simulink model "EReg_Tank_Drainrefusestowork"  (R2025b)
settings: Solver=FixedStepAuto  StartTime=0.0  StopTime=Sim_Duration  FixedStep=1/500  RelTol=1e-3
values from neighbouring files (symbols this model uses):
  A_3 = 13.27e-6    (= 1.327e-05)    [EReg_N2O_Simulink_Init.m]    (also in EReg_Tank_Drain_Init.m = 6e-05)
  Cd_3 = 0.6    [EReg_N2O_Simulink_Init.m]    (also in EReg_Tank_Drain_Init.m = 0.7)
  gamma_N2 = 1.4    [EReg_N2O_Simulink_Init.m]    (also in EReg_Tank_Drain_Init.m; EReg_Tank_Drain_N2O_Sim.m; N2O_Tank_Plant.m)
  K_v_4 = 0.5    [EReg_Tank_Drain_Init.m]
  Kv_1_max = 1.5    [EReg_N2O_Simulink_Init.m]    (also in EReg_Tank_Drain_Init.m = 1; EReg_Tank_Drain_N2O_Sim.m = params.Kv_1_max)
  m_1_0 = rho_1_0 * V_1    (= 2.35097796073)    [EReg_N2O_Simulink_Init.m]    (also in EReg_Tank_Drain_Init.m = 2.2972972973; EReg_Tank_Drain_N2O_Sim.m = params.m_1_0)
  m_2_0 = m_N2_ull_0    [EReg_N2O_Simulink_Init.m]    (also in EReg_Tank_Drain_Init.m = 0.281531531532)
  m_3_0 = m_N2O_liq_0    (= 12)    [EReg_N2O_Simulink_Init.m]    (also in EReg_Tank_Drain_Init.m = 20)
  P_1_0 = 300e5    (= 30000000)    [EReg_N2O_Simulink_Init.m]    (also in EReg_Tank_Drain_Init.m; EReg_Tank_Drain_N2O_Sim.m = params.P_1_0)
  Pst = 101325    [EReg_N2O_Simulink_Init.m]    (also in EReg_Tank_Drain_Init.m)
  R_N2 = 296    [EReg_N2O_Simulink_Init.m]    (also in EReg_Tank_Drain_Init.m; EReg_Tank_Drain_N2O_Sim.m = params.R_N2)
  rho_1_0 = P_1_0 / (R_N2 * T_0_N2)    (= 345.732053049)    [EReg_N2O_Simulink_Init.m]    (also in EReg_Tank_Drain_Init.m = 337.837837838; EReg_Tank_Drain_N2O_Sim.m = m_1_0 / V_1)
  rho_L = rhoL_init    [EReg_N2O_Simulink_Init.m]    (also in EReg_Tank_Drain_Init.m = 1000; EReg_Tank_Drain_N2O_Sim.m = T_to_rhoL(T); EregPlot.m = 1000; N2O_Tank_Plant.m = interp1_lut(T_sat_LUT, rhoL_LUT, T_N2O))
  rhost = Pst / (R_N2 * Tst)    (= 1.25320955222)    [EReg_N2O_Simulink_Init.m]    (also in EReg_Tank_Drain_Init.m)
  servo_off_setpoint = ones(1, Num_Steps)    [EReg_N2O_Simulink_Init.m]    (also in EReg_Tank_Drain_Init.m = zeros(1, Num_Steps))
  T_0_N2 = 293.15    [EReg_N2O_Simulink_Init.m]    (also in EReg_Tank_Drain_Init.m = 300)
  time = linspace(0, Sim_Duration, Num_Steps)    [EReg_N2O_Simulink_Init.m]    (also in EReg_Tank_Drain_Init.m; EReg_Tank_Drain_N2O_Sim.m = (0 : dt : t_end)')
  Tst = 273.15    [EReg_N2O_Simulink_Init.m]    (also in EReg_Tank_Drain_Init.m)
  V_1 = 6.8e-3    (= 0.0068)    [EReg_N2O_Simulink_Init.m]    (also in EReg_Tank_Drain_Init.m; EReg_Tank_Drain_N2O_Sim.m = params.V_1)
  V_2 = 30e-3    (= 0.03)    [EReg_N2O_Simulink_Init.m]    (also in EReg_Tank_Drain_Init.m = 0.025; EReg_Tank_Drain_N2O_Sim.m = params.V_2)
undefined symbols (not defined in the file or in its folder): DiscIntNeverNeededParam
libraries: simulink x2, slpidlib x1
settings Model: Creator=marti  LastModifiedBy=anzashoaib
settings OptimizationCC: ReuseModelBlockBuffer=off
settings RTWCC: GPUComputeCapability=3.5

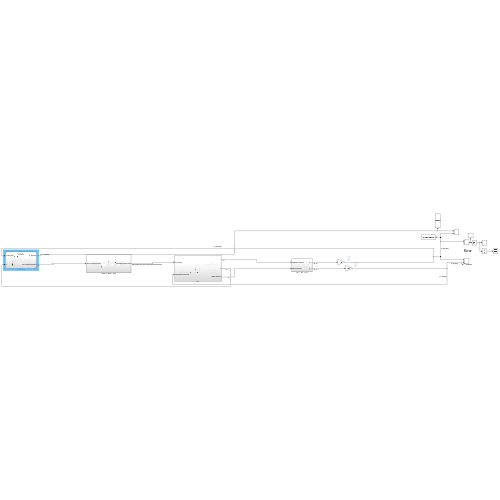
[thumbnail: Simulink's stored preview of the top-level diagram]
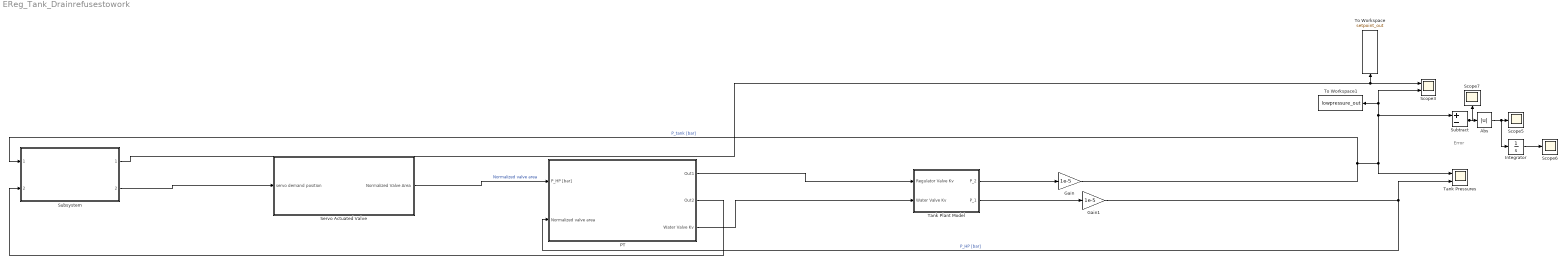
== system EReg_Tank_Drainrefusestowork ==
  note: Error
  Abs : Abs  SaturateOnIntegerOverflow=off
  Gain : Gain  Gain=1e-5
  Gain1 : Gain  Gain=1e-5
  Integrator : Integrator
  "PT " : Subsystem
  Scope3 : Scope  NumInputPorts=2
      settings: ActiveDisplayYMinimum=51.75312  ActiveDisplayYMaximum=64.23854
  Scope5 : Scope
      settings: ActiveDisplayYMinimum=-0.46907  ActiveDisplayYMaximum=4.2216
  Scope6 : Scope
      settings: ActiveDisplayYMinimum=-42.4732  ActiveDisplayYMaximum=382.25884  DataLoggingVariableName=ScopeData2
  Scope7 : Scope
      settings: ActiveDisplayYMinimum=-4.72126  ActiveDisplayYMaximum=4.96726  DataLoggingVariableName=ScopeData3
  Servo Actuated Valve : Subsystem
  Subsystem : Subsystem  ReferencedSubsystem=Controller
  Subtract : Sum  Inputs=+-
  Tank Plant Model : Subsystem
  Tank Pressures : Scope  NumInputPorts=2
      settings: ActiveDisplayYMinimum=22.037093774647268  ActiveDisplayYMaximum=330.88476735837253
  To Workspace : ToWorkspace  VariableName=setpoint_out  SaveFormat=Timeseries  SampleTime=-1
  To Workspace1 : ToWorkspace  VariableName=lowpressure_out  SaveFormat=Timeseries  SampleTime=-1
  wires:
  Tank Plant Model/1(P_2) -> Gain/1
  Tank Plant Model/2(P_1) -> Gain1/1
  Gain/1 -> Subsystem/1, Subtract/1, Scope3/2, To Workspace1/1, Tank Pressures/1  "P_tank [bar]"
  Gain1/1 -> "PT "/2(Normalized valve area), Tank Pressures/2  "P_HP [bar]"
  Subtract/1 -> Scope7/1, Abs/1
  Abs/1 -> Integrator/1, Scope5/1
  Integrator/1 -> Scope6/1
  Subsystem/1 -> To Workspace/1, Scope3/1
  Subsystem/2 -> Servo Actuated Valve/1(servo demand position)
  Servo Actuated Valve/1(Normalized Valve Area) -> "PT "/1(P_HP [bar])  "Normalized valve area"
  "PT "/1(Out1) -> Tank Plant Model/1(Regulator Valve Kv)
  "PT "/2(Out2) -> Subsystem/2
  "PT "/3(Water Valve Kv) -> Tank Plant Model/2(Water Valve Kv)

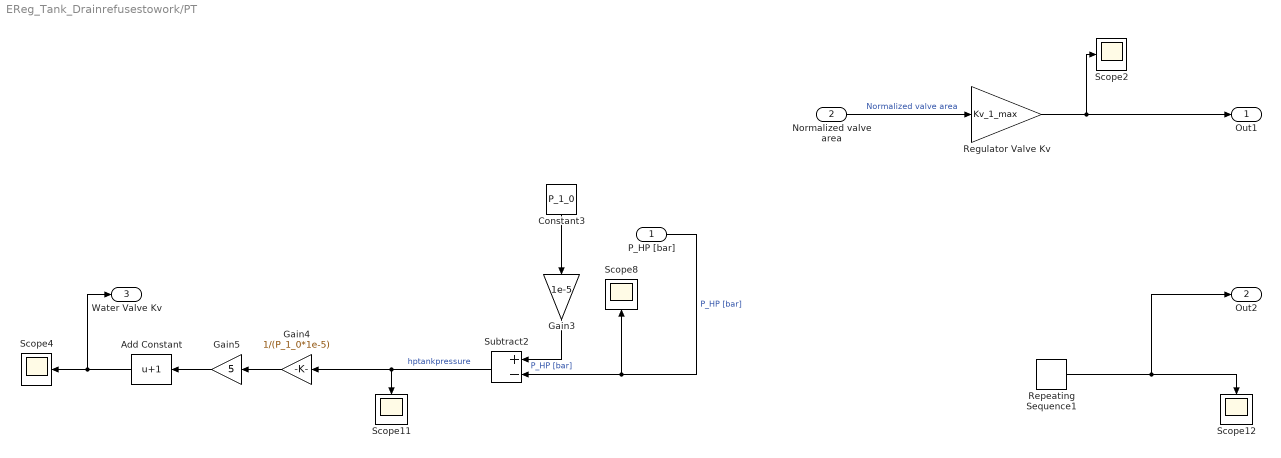
== system EReg_Tank_Drainrefusestowork/PT  ==
  P_HP [bar] : Inport  OutDataTypeStr=double  PortDimensions=1  SampleTime=0
  Normalized valve area : Inport  Port=2  OutDataTypeStr=double  PortDimensions=1  SampleTime=0
  Add Constant : Bias  Bias=1  SaturateOnIntegerOverflow=off
  Constant3 : Constant  Value=P_1_0
  Gain3 : Gain  Gain=1e-5
  Gain4 : Gain  Gain=1/(P_1_0*1e-5)
  Gain5 : Gain  Gain=5
  Regulator Valve Kv : Gain  Gain=Kv_1_max
  Repeating Sequence1 : simulink/Sources/Repeating Sequence  rep_seq_t=time  rep_seq_y=run_valve_setpoint
  Scope{2,4,8,11..12} (5 alike) : Scope
      Scope11 settings: ActiveDisplayYMinimum=-7.98984  ActiveDisplayYMaximum=71.90855  DataLoggingVariableName=ScopeData15
      Scope12 settings: ActiveDisplayYMinimum=-0.125  ActiveDisplayYMaximum=1.125  DataLoggingVariableName=ScopeData16
      Scope2 settings: ActiveDisplayYMinimum=-0.0196  ActiveDisplayYMaximum=0.17636  DataLoggingVariableName=ScopeData17
      Scope4 settings: ActiveDisplayYMinimum=0.86684  ActiveDisplayYMaximum=2.19848  DataLoggingVariableName=ScopeData18
      Scope8 settings: ActiveDisplayYMinimum=229.43787  ActiveDisplayYMaximum=307.84024  DataLoggingVariableName=ScopeData19
  Subtract2 : Sum  Inputs=+-
  Out1 : Outport  OutDataTypeStr=double  PortDimensions=1  SampleTime=0
  Out2 : Outport  Port=2  OutDataTypeStr=double  PortDimensions=1  SampleTime=0
  Water Valve Kv : Outport  Port=3  OutDataTypeStr=double  PortDimensions=1  SampleTime=0
  wires:
  Add Constant/1 -> Water Valve Kv/1, Scope4/1
  Gain3/1 -> Subtract2/1  "P_HP [bar]"
  Gain4/1 -> Gain5/1
  Repeating Sequence1/1 -> Scope12/1, Out2/1
  P_HP [bar]/1 -> Scope8/1, Subtract2/2  "P_HP [bar]"
  Regulator Valve Kv/1 -> Out1/1, Scope2/1
  Constant3/1 -> Gain3/1
  Subtract2/1 -> Gain4/1, Scope11/1  "hptankpressure"
  Gain5/1 -> Add Constant/1
  Normalized valve area/1 -> Regulator Valve Kv/1  "Normalized valve area"

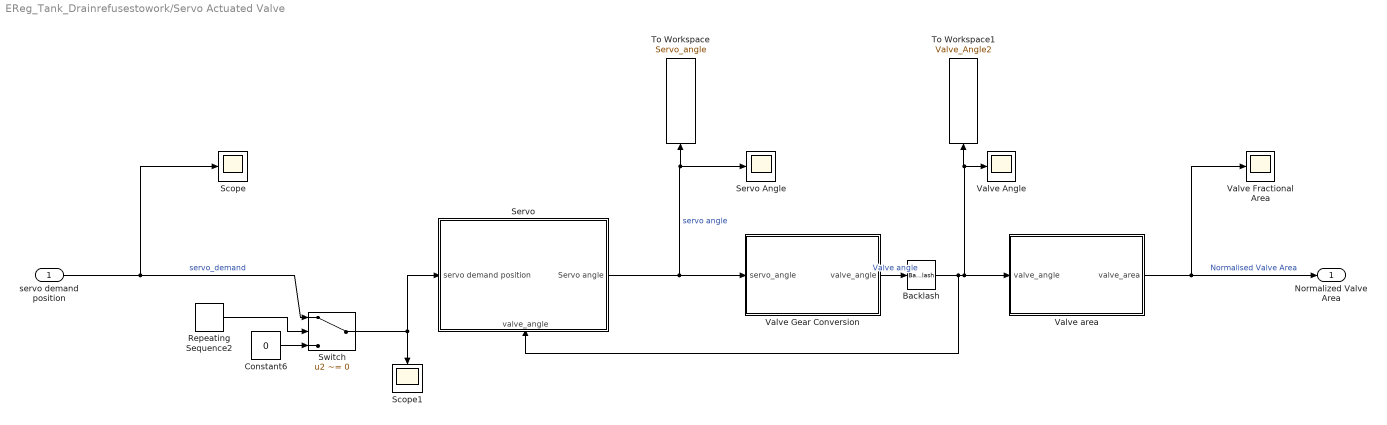
== system EReg_Tank_Drainrefusestowork/Servo Actuated Valve ==
  servo demand position : Inport
  " Valve Gear Conversion" : MATLAB Function  TreatAsAtomicUnit=on
  " Valve area" : MATLAB Function  TreatAsAtomicUnit=on
  Backlash : Backlash  BacklashWidth=0.5  InitialOutput=0.5
  Constant6 : Constant  Value=0
  Repeating Sequence2 : simulink/Sources/Repeating Sequence  rep_seq_t=time(:)  rep_seq_y=servo_off_setpoint(:)
  Scope : Scope
      settings: ActiveDisplayYMinimum=-1660.50954  ActiveDisplayYMaximum=362.9195  DataLoggingVariableName=ScopeData3
  Scope1 : Scope
      settings: ActiveDisplayYMinimum=-1660.50954  ActiveDisplayYMaximum=362.9195  DataLoggingVariableName=ScopeData3
  Servo : Subsystem
      settings: PortSchema="{\"entries\":[{\"content\":{\"sides\":[{\"content\":{\"connectorIds\":[\"In1\"]},\"type\":\"ConnectorPlacement.EquallySpacedRectSide\",\"uuid\":\"80cc8390-5c54-44fd-a47c-7e7786ca55cb\"},{\"content\":{\"connectorIds\":[\"Out1\"],\"side\":\"RIGHT\"},\"type\":\"ConnectorPlacement.EquallySpacedRectSide\",\"uuid\":\"1eac09ca-847a-4c9b-93fa-12e39acf6b4a\"},{\"content\":{\"side\":\"TOP\"},\"type\":\"ConnectorPlacement.EquallySpacedRectSide\",\"uuid\":\"448ec877-4708-4b6f-bd0d-b7e31e141685\"},{\"content\":{\"connectorIds\":[\"In2\"],\"side\":\"BOTTOM\"},\"type\":\"ConnectorPlacement.EquallySpacedRectSide\",\"uuid\":\"b9bb9fb8-2143-4f55-8173-037b619887c5\"}]},\"type\":\"ConnectorPlacement.EquallySpacedConnector\",\"uuid\":\"bf70c898-a427-4eb9-a0e2-218e58098715\"}],\"packageUris\":[\"http://schema.mathworks.com/mf0/Connector/R2020b\"],\"version\":\"1.0\"}"
  Servo Angle : Scope
      settings: ActiveDisplayYMinimum=-2.83907  ActiveDisplayYMaximum=21.23036  DataLoggingVariableName=Servo_Angle  DataLoggingSaveFormat=Array
  Switch : Switch  Criteria=u2 ~= 0  SaturateOnIntegerOverflow=off  InputSameDT=off
  To Workspace : ToWorkspace  VariableName=Servo_angle  SampleTime=-1
      settings: Save2DSignal=2-D array (concatenate along first dimension)
  To Workspace1 : ToWorkspace  VariableName=Valve_Angle2  SampleTime=-1
      settings: Save2DSignal=2-D array (concatenate along first dimension)
  Valve Angle : Scope
      settings: ActiveDisplayYMinimum=-1.35754  ActiveDisplayYMaximum=12.17595  DataLoggingVariableName=Valve_Angle  DataLoggingSaveFormat=Array
  Valve Fractional Area : Scope
      settings: ActiveDisplayYMinimum=-0.0196  ActiveDisplayYMaximum=0.17636  DataLoggingVariableName=ScopeData8
  Normalized Valve Area : Outport
  wires:
  " Valve area"/1(valve_area) -> Normalized Valve Area/1, Valve Fractional Area/1  "Normalised Valve Area"
  " Valve Gear Conversion"/1(valve_angle) -> Backlash/1  "Valve angle"
  servo demand position/1 -> Scope/1, Switch/1  "servo_demand"
  Servo/1(Servo angle) -> " Valve Gear Conversion"/1(servo_angle), To Workspace/1, Servo Angle/1  "servo angle"
  Repeating Sequence2/1 -> Switch/2
  Constant6/1 -> Switch/3
  Switch/1 -> Servo/1(servo demand position), Scope1/1
  Backlash/1 -> " Valve area"/1(valve_angle), To Workspace1/1, Valve Angle/1, Servo/2(valve_angle)

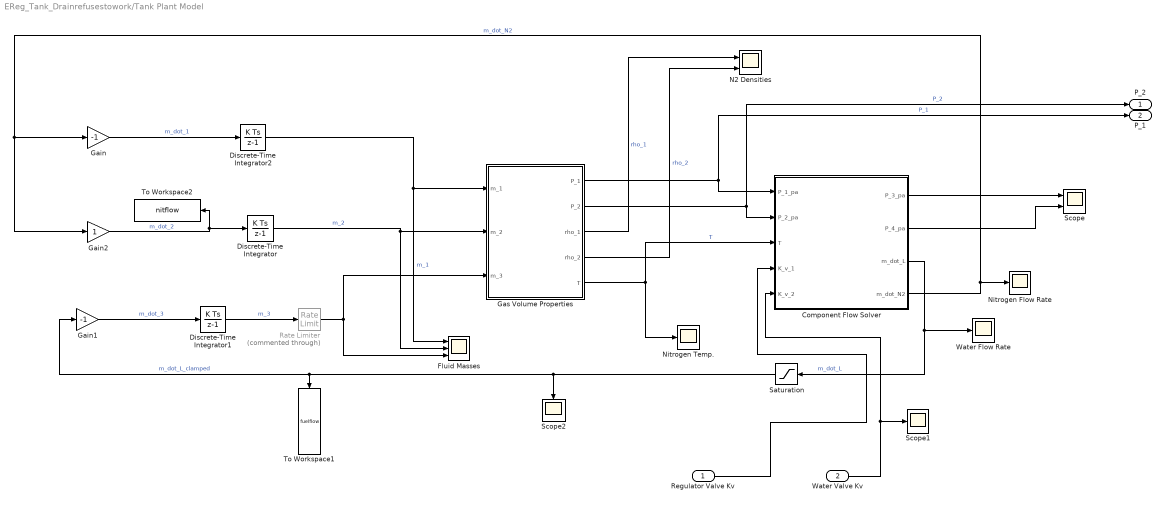
== system EReg_Tank_Drainrefusestowork/Tank Plant Model ==
  Regulator Valve Kv : Inport
  Water Valve Kv : Inport  Port=2
  Component Flow Solver : MATLAB Function  TreatAsAtomicUnit=on
  Discrete-Time Integrator : DiscreteIntegrator  InitialCondition=m_2_0  SampleTime=-1  ICPrevOutput=DiscIntNeverNeededParam  ICPrevScaledInput=DiscIntNeverNeededParam
  Discrete-Time Integrator1 : DiscreteIntegrator  InitialCondition=m_3_0  SampleTime=-1  ICPrevOutput=DiscIntNeverNeededParam  ICPrevScaledInput=DiscIntNeverNeededParam
  Discrete-Time Integrator2 : DiscreteIntegrator  InitialCondition=m_1_0  SampleTime=-1  ICPrevOutput=DiscIntNeverNeededParam  ICPrevScaledInput=DiscIntNeverNeededParam
  Fluid Masses : Scope  NumInputPorts=3
      settings: ActiveDisplayYMinimum=-0.63894  ActiveDisplayYMaximum=8.95988  DataLoggingVariableName=ScopeData4
  Gain : Gain  Gain=-1
  Gain1 : Gain  Gain=-1
  Gain2 : Gain
  Gas Volume Properties : MATLAB Function  TreatAsAtomicUnit=on
  N2 Densities : Scope  NumInputPorts=2
      settings: ActiveDisplayYMinimum=-3.2542  ActiveDisplayYMaximum=338.19949  DataLoggingVariableName=ScopeData5
  Nitrogen Flow Rate : Scope
      settings: ActiveDisplayYMinimum=-0.0436  ActiveDisplayYMaximum=0.39242  DataLoggingVariableName=ScopeData2
  Nitrogen Temp. : Scope
      settings: ActiveDisplayYMinimum=261.34234  ActiveDisplayYMaximum=304.2953  DataLoggingVariableName=ScopeData3
  Rate Limiter : RateLimiter  Commented=through  RisingSlewLimit=0  FallingSlewLimit=-999999999  SampleTimeMode=inherited
  Saturation : Saturate  UpperLimit=inf  LowerLimit=0
  Scope : Scope  NumInputPorts=2
      settings: ActiveDisplayYMinimum=-1.77844825772E+6  ActiveDisplayYMaximum=1.600603055574E+7  DataLoggingVariableName=ScopeData6
  Scope1 : Scope
      settings: ActiveDisplayYMinimum=-0.125  ActiveDisplayYMaximum=1.125
  Scope2 : Scope
      settings: ActiveDisplayYMinimum=-0.23736  ActiveDisplayYMaximum=2.13625  DataLoggingVariableName=ScopeData2
  To Workspace1 : ToWorkspace  VariableName=fuelflow  SaveFormat=Timeseries  SampleTime=-1
  To Workspace2 : ToWorkspace  VariableName=nitflow  SaveFormat=Timeseries  SampleTime=-1
  Water Flow Rate : Scope
      settings: ActiveDisplayYMinimum=-0.17675  ActiveDisplayYMaximum=1.59071
  P_2 : Outport
  P_1 : Outport  Port=2
  wires:
  Gas Volume Properties/1(P_1) -> P_1/1, Component Flow Solver/1(P_1_pa)  "P_1"
  Gain/1 -> Discrete-Time Integrator2/1  "m_dot_1"
  Component Flow Solver/1(P_3_pa) -> Scope/1
  Discrete-Time Integrator/1 -> Fluid Masses/2, Gas Volume Properties/2(m_2)  "m_2"
  Discrete-Time Integrator2/1 -> Fluid Masses/1, Gas Volume Properties/1(m_1)  "m_1"
  Component Flow Solver/2(P_4_pa) -> Scope/2
  Gain1/1 -> Discrete-Time Integrator1/1  "m_dot_3"
  Component Flow Solver/4(m_dot_N2) -> Nitrogen Flow Rate/1, Gain2/1, Gain/1  "m_dot_N2"
  Gain2/1 -> Discrete-Time Integrator/1, To Workspace2/1  "m_dot_2"
  Discrete-Time Integrator1/1 -> Rate Limiter/1  "m_3"
  Gas Volume Properties/2(P_2) -> P_2/1, Component Flow Solver/2(P_2_pa)  "P_2"
  Component Flow Solver/3(m_dot_L) -> Saturation/1, Water Flow Rate/1  "m_dot_L"
  Gas Volume Properties/4(rho_2) -> N2 Densities/2  "rho_2"
  Gas Volume Properties/3(rho_1) -> N2 Densities/1  "rho_1"
  Gas Volume Properties/5(T) -> Nitrogen Temp./1, Component Flow Solver/3(T)  "T"
  Water Valve Kv/1 -> Scope1/1, Component Flow Solver/5(K_v_2)
  Regulator Valve Kv/1 -> Component Flow Solver/4(K_v_1)
  Rate Limiter/1 -> Gas Volume Properties/3(m_3), Fluid Masses/3
  Saturation/1 -> Scope2/1, To Workspace1/1, Gain1/1  "m_dot_L_clamped"

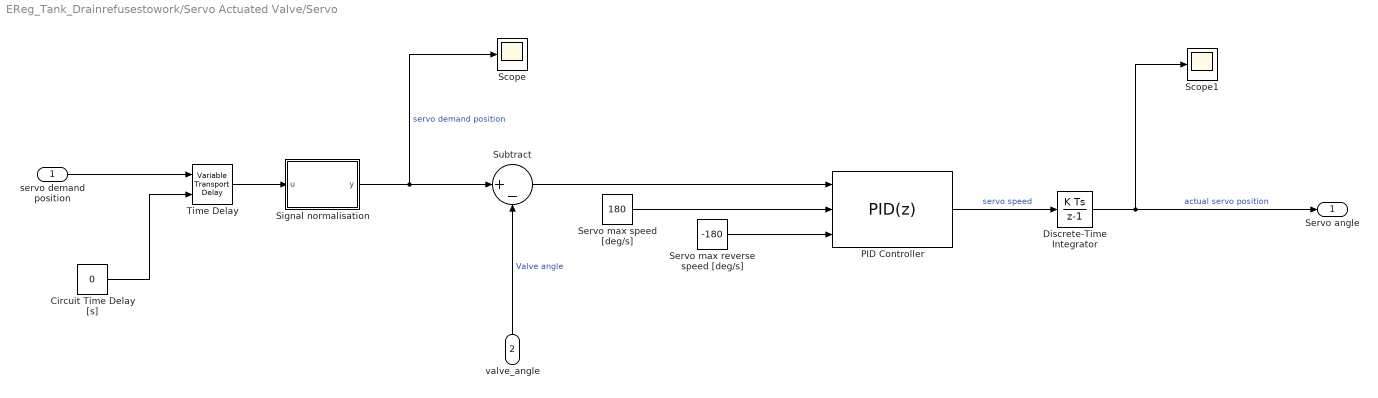
== system EReg_Tank_Drainrefusestowork/Servo Actuated Valve/Servo ==
  servo demand position : Inport
  valve_angle : Inport  Port=2
  Circuit Time Delay [s] : Constant  Value=0
  Discrete-Time Integrator : DiscreteIntegrator  SampleTime=-1  ICPrevOutput=DiscIntNeverNeededParam  ICPrevScaledInput=DiscIntNeverNeededParam
  PID Controller : slpidlib/PID Controller  Controller=PID  Form=Parallel  TimeDomain=Discrete-time  UseExternalTs=off  SampleTime=-1  IntegratorMethod=Forward Euler  FilterMethod=Forward Euler  ControllerParametersSource=internal  P=3  I=2  UseKiTs=off  D=0  UseExternalDerivativeSource=off  N=100  UseFilter=on  TunerSelectOption=Transfer Function Based (PID Tuner App)  InitialConditionSource=internal  InitialConditionForIntegrator=0  InitialConditionForFilter=0  DifferentiatorICPrevScaledInput=0  ExternalReset=none  TrackingMode=off  Kt=1  LimitOutput=on  SatLimitsSource=external  UpperSaturationLimit=inf  LowerSaturationLimit=-inf  LinearizeAsGain=on  AntiWindupMode=none  Kb=1  LimitIntegrator=off  UpperIntegratorSaturationLimit=inf  LowerIntegratorSaturationLimit=-inf  POutMin=[]  POutMax=[]  IOutMin=[]  IOutMax=[]  DOutMin=[]  DOutMax=[]  NOutMin=[]  NOutMax=[]  SumOutMin=[]  SumOutMax=[]  SaturationOutMin=[]  SaturationOutMax=[]  PParamMin=[]  PParamMax=[]  IParamMin=[]  IParamMax=[]  DParamMin=[]  DParamMax=[]  NParamMin=[]  NParamMax=[]  KbParamMin=[]  KbParamMax=[]  KtParamMin=[]  KtParamMax=[]  KbOutMin=[]  KbOutMax=[]  KtOutMin=[]  KtOutMax=[]  IntegratorOutMin=[]  IntegratorOutMax=[]  FilterOutMin=[]  FilterOutMax=[]  SumI1OutMin=[]  SumI1OutMax=[]  SumI2OutMin=[]  SumI2OutMax=[]  SumI3OutMin=[]  SumI3OutMax=[]  SumI4OutMin=[]  SumI4OutMax=[]  SumDOutMin=[]  SumDOutMax=[]  DifferentiatorOutMin=[]  DifferentiatorOutMax=[]  FilterDiffOutCoefMin=[]  FilterDiffOutCoefMax=[]  ReciprocalOutMin=[]  ReciprocalOutMax=[]  SumDenOutMin=[]  SumDenOutMax=[]  SumNumOutMin=[]  SumNumOutMax=[]  DivideOutMin=[]  DivideOutMax=[]  UdiffTsProdOutMin=[]  UdiffTsProdOutMax=[]  NTsProdOutMin=[]  NTsProdOutMax=[]  UintegralTsProdOutMin=[]  UintegralTsProdOutMax=[]  UngainTsProdOutMin=[]  UngainTsProdOutMax=[]  ClampingZeroOutDataTypeStr=Inherit: Inherit via back propagation  ClampingZeroOutMin=[]  ClampingZeroOutMax=[]  FilterDenConstantOutDataTypeStr=Inherit: Inherit via back propagation  FilterDenConstantOutMin=[]  FilterDenConstantOutMax=[]  PCopyOutDataTypeStr=Inherit: Inherit via back propagation  PCopyOutMin=[]  PCopyOutMax=[]  NCopyOutDataTypeStr=Inherit: Inherit via back propagation  NCopyOutMin=[]  NCopyOutMax=[]  IntegratorContinuousStateAttributes=''  IntegratorStateMustResolveToSignalObject=off  IntegratorRTWStateStorageClass=Auto  FilterContinuousStateAttributes=''  FilterStateMustResolveToSignalObject=off  FilterRTWStateStorageClass=Auto  ParallelPVariant=InternalParameters  IdealPVariant=Disabled  IVariant=InternalParameters  DVariant=InternalParameters  IntegratorVariant=Discrete  SatVariant=External  AWVariant=Passthrough  PCopyVariant=Disabled  TRVariant=Disabled  FdbkBlocksVariant=Forward  IdealPFdbkVariant=Disabled  SatFdbkVariant=Disabled  DerivativeFilterVariant=ForwardEulerFilter  NVariant=InternalParameters  NCopyVariant=Disabled  FilterICVariant=InternalICsFilter  IntegratorICVariant=InternalICs  ExternalResetVariant=Disabled  TRSumVariant=Passthrough  SumFdbkVariant=Disabled  SumVariant=Sum_PID  TsampFilterVariant=InternalTs  TsampNgainVariant=Passthrough  TsampIntegralVariant=Disabled_SignalSpec  ExternalSaturationOutDataTypeStr=Inherit: Same as second input  DerivativeSourceVariant=ErrorSignal  PreIntVariant=InternalPreInt
  Scope : Scope
      settings: ActiveDisplayYMinimum=-20.07207  ActiveDisplayYMaximum=180.64867
  Scope1 : Scope
      settings: ActiveDisplayYMinimum=-2.83907  ActiveDisplayYMaximum=21.23036  DataLoggingVariableName=ScopeData2
  Servo max reverse speed [deg/s] : Constant  Value=-180
  Servo max speed [deg/s] : Constant  Value=180
  Signal normalisation : MATLAB Function  TreatAsAtomicUnit=on
  Subtract : Sum  Inputs=|+-
  Time Delay : VariableTransportDelay  MaximumDelay=10  MaximumPoints=6000  ZeroDelay=on
  Servo angle : Outport
  wires:
  Servo max reverse speed [deg/s]/1 -> PID Controller/3
  Servo max speed [deg/s]/1 -> PID Controller/2
  PID Controller/1 -> Discrete-Time Integrator/1  "servo speed"
  Discrete-Time Integrator/1 -> Scope1/1, Servo angle/1  "actual servo position"
  Subtract/1 -> PID Controller/1
  Signal normalisation/1(y) -> Scope/1, Subtract/1  "servo demand position"
  servo demand position/1 -> Time Delay/1
  Time Delay/1 -> Signal normalisation/1(u)
  Circuit Time Delay [s]/1 -> Time Delay/2
  valve_angle/1 -> Subtract/2  "Valve angle"

== matlab function EReg_Tank_Drainrefusestowork/Tank Plant Model/Component Flow Solver ==
  data: P_1_pa input; P_2_pa input; P_3_pa output; T input; P_4_pa output; m_dot_L output; m_dot_N2 output; K_v_1 input; K_v_2 input; Cd_3 parameter; K_v_4 parameter; rho_L parameter; R_N2 parameter; Tst parameter; rhost parameter; A_3 parameter; Pst parameter
function [P_3_pa, P_4_pa, m_dot_L, m_dot_N2] = fcn(P_1_pa, P_2_pa, T, K_v_1, K_v_2, Cd_3, K_v_4, rho_L, R_N2, Tst, rhost, A_3, Pst)
%#codegen

% This function solves for the intermediate pressures and mass flows in a
% fluid system. It replaces a non-codegen-compatible 'fsolve' call with
% two independent 1D Newton-Raphson solvers.

% --- Solver Parameters ---
MAX_ITER = 50;  % Maximum iterations for Newton's method
TOLERANCE = 1e-7; % Convergence tolerance
h = 1e-6;       % Step size for numerical derivative
P_atm_pa = 101325;
% --- Input Conversions ---
% Convert input pressures from Pascals (pa) to bar for K_v calcs
P_1 = P_1_pa * 1e-5;
P_2 = P_2_pa * 1e-5;
% Note: P_atm_pa is passed directly to calc_m_dot_b, which expects Pascals

% --- Problem Setup ---
% Calculate Specific Gravity for liquid flow
SG = rho_L / 1000.0;

% --- 1. Solve for Liquid-Side Pressure P_3 ---
% We need to find P_3 (in bar) such that: liquid_error(P_3) = 0
% where liquid_error = calc_m_dot_a(P_3) - calc_m_dot_b(P_3)

% Define the error function for the liquid side
% All parameters are passed anonymously
liquid_error_fun = @(p3) (calc_m_dot_a(p3, P_2, K_v_2, rho_L, SG) - ...
                          calc_m_dot_b(p3, Cd_3, A_3, rho_L, P_atm_pa));

% Initial guess for P_3 (in bar)
x0_P3 = 1.0; 

% Call the Newton solver
P_3_bar = newton_solver(liquid_error_fun, x0_P3, MAX_ITER, TOLERANCE, h);

% --- 2. Solve for Gas-Side Pressure P_4 ---
% We need to find P_4 (in bar) such that: gas_error(P_4) = 0
% where gas_error = calc_m_dot_c(P_4) - calc_m_dot_d(P_4)

% Define the error function for the gas side
gas_error_fun = @(p4) (calc_m_dot_c(p4, P_1, K_v_1, rhost, T, Pst, R_N2, Tst) - ...
                       calc_m_dot_d(p4, P_2, K_v_4, rhost, T, Pst, R_N2, Tst));
                       
% Initial guess for P_4 (in bar)
x0_P4 = 1.0; 

% Call the Newton solver
P_4_bar = newton_solver(gas_error_fun, x0_P4, MAX_ITER, TOLERANCE, h);

% --- 3. Calculate Final Outputs ---
% Convert pressures back to Pascals
P_3_pa = P_3_bar * 1e5;
P_4_pa = P_4_bar * 1e5;

% Calculate the final mass flow rates using the solved pressures
m_dot_L  = calc_m_dot_a(P_3_bar, P_2, K_v_2, rho_L, SG);
m_dot_N2 = calc_m_dot_c(P_4_bar, P_1, K_v_1, rhost, T, Pst, R_N2, Tst);

end

% =========================================================================
% --- NESTED HELPER FUNCTIONS (CODEGEN-COMPATIBLE) ---
% =========================================================================

function x_root = newton_solver(fun, x0, max_iter, tol, h)
% A simple 1D Newton-Raphson solver using a numerical derivative.
% It finds x such that fun(x) = 0.
    
    x_root = x0;
    for i = 1:max_iter
        % Calculate function value at current point
        f_val = fun(x_root);
        
        % Check for convergence
        if abs(f_val) < tol
            return; % Solution found
        end
        
        % Calculate function value at a small step h away
        f_val_h = fun(x_root + h);
        
        % Calculate numerical derivative (Jacobian)
        f_deriv = (f_val_h - f_val) / h;
        
        % Check for division by zero (flat gradient)
        if abs(f_deriv) < 1e-10
            % Cannot converge, return last best guess
            return;
        end
        
        % Newton's step
        x_new = x_root - f_val / f_deriv;
        
        % Check for step convergence
        if abs(x_new - x_root) < tol
            x_root = x_new;
            return; % Solution found
        end
        
        x_root = x_new;
    end
    % If loop finishes, max iterations were reached. Return last value.
end


function m_dot_a = calc_m_dot_a(P_3, P_2, K_v_2, rho_L, SG)
% Water Control Valve (m_dot_a)
% All pressures in bar
    delta_P = P_2 - P_3;
    % Use sign(delta_P) to handle potential flow reversal safely
    Q = K_v_2 * (delta_P / SG) / sqrt(abs(delta_P / SG) + 1e-9); 
    m_dot_a = Q * rho_L * (1/3600); % Convert standard flow rate to mass flow rate
end


function m_dot_b = calc_m_dot_b(P_3_bar, Cd_3, A_3, rho_L, P_atm_pa)
% Water Orifice (m_dot_b)
% P_3_bar is in bar, P_atm_pa is in Pascals
    
    % Convert P_3 from bar to Pascals for this equation
    P_3_pa = P_3_bar * 1e5;
    delta_P_pa = P_3_pa - P_atm_pa;
    
    % This formulation from your original code correctly handles flow
    % direction using sign(delta_P) * sqrt(abs(delta_P))
    m_dot_b = Cd_3 * A_3 * 2 * rho_L * delta_P_pa / sqrt(abs(2 * rho_L * delta_P_pa) + 1e-9);
end


function m_dot_c = calc_m_dot_c(P_4, P_1, K_v_1, rhost, T, Pst, R_N2, Tst)
% Regulator Valve (m_dot_c)
% All pressures in bar
    Q_N = 0.0;
    if (P_4 >= 0.528 * P_1)
        % Non-choked flow
        arg = (P_1 - P_4) * P_4 / (rhost * T);
        Q_N = K_v_1 * 514 * arg / sqrt(abs(arg) + 1e-9);
    else
        % Choked flow
        Q_N = K_v_1 * 257 * P_1 / sqrt(abs(rhost * T) + 1e-9);
    end
    m_dot_c = Q_N * (Pst / (R_N2 * Tst)) * (1/3600); % Convert standard flow rate to mass flow rate
end


function m_dot_d = calc_m_dot_d(P_4, P_2, K_v_4, rhost, T, Pst, R_N2, Tst)
% Check Valve (m_dot_d)
% All pressures in bar
    Q_N = 0.0;
    if (P_2 >= 0.528 * P_4)
        % Non-choked flow
        arg = (P_4 - P_2) * P_2 / (rhost * T);
        Q_N = K_v_4 * 514 * arg / sqrt(abs(arg) + 1e-9);
    else
        % Choked flow
        Q_N = K_v_4 * 257 * P_4 / sqrt(abs(rhost * T) + 1e-9);
    end
    m_dot_d = Q_N * (Pst / (R_N2 * Tst)) * (1/3600); % Convert standard flow rate to mass flow rate
end

== matlab function EReg_Tank_Drainrefusestowork/Tank Plant Model/Gas Volume Properties ==
  data: P_1 output; P_2 output; m_1 input; rho_1 output; m_2 input; m_3 input; rho_2 output; T output; V_1 parameter; V_2 parameter; T_0_N2 parameter; rho_1_0 parameter; gamma_N2 parameter; R_N2 parameter; rho_L parameter
function [P_1, P_2, rho_1, rho_2, T]= fcn(m_1, m_2, m_3, V_1, V_2, T_0_N2, rho_1_0, gamma_N2, R_N2, rho_L)

rho_1 = m_1/V_1; %Find the HP tank gas density
rho_2 = m_2/(V_2 - m_3/rho_L); %Find the ullage gas density
T = T_0_N2*(rho_1/rho_1_0)^(gamma_N2 - 1); %Find the ullage gas temperature (assumiong adiabatic expansion)
P_1 = rho_1*R_N2*T; %Find the HP gas pressure
P_2 = rho_2*R_N2*T; %Find the ullage gas pressure (Tank pressure)

== matlab function EReg_Tank_Drainrefusestowork/Servo Actuated Valve/ Valve Gear Conversion ==
  data: servo_angle input; valve_angle output
function valve_angle = fcn(servo_angle)

valve_angle = servo_angle/1.7; % check gear ratio with oscar
%valve_angle = servo_angle;

== matlab function EReg_Tank_Drainrefusestowork/Servo Actuated Valve/ Valve area ==
  data: valve_angle input; valve_area output
function valve_area = fcn(valve_angle)
valve_angle = valve_angle - 5; %Account for first part of rotation where valve doesn't open at all
if valve_angle < 0
    valve_area = 0;
else
    valve_area = 1.1*((5*10^-6)*valve_angle^3 - 0.0006*valve_angle^2 + 0.0278*valve_angle); %calculate normalised valve area
end

== matlab function EReg_Tank_Drainrefusestowork/Servo Actuated Valve/Servo/Signal normalisation ==
  data: u input; y output
function y = fcn(u)
if u < 0
    y = 0;
else 
    if u > 180
        y = 180;
    else
        y = u;
    end
end
